simulink model "MultiUser_Model"  (R2016b)
settings: Solver=VariableStepAuto  StartTime=0.0  StopTime=inf  RelTol=1e-3
PreLoadFcn:
  | try, eval([bdroot '_setup']); catch, eval('MultiUser_setup', ''); end
libraries: MultiUser_Lib x3
settings Model: Creator=HP  LastModifiedBy=HP

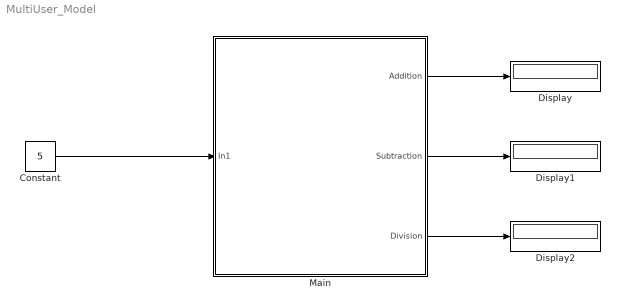
== system MultiUser_Model ==
  Constant : Constant  Value=5
  Display : Display
  Display1 : Display
  Display2 : Display
  Main : Subsystem
  wires:
  Constant/1 -> Main/1(In1)
  Main/1(Addition) -> Display/1
  Main/2(Subtraction) -> Display1/1
  Main/3(Division) -> Display2/1

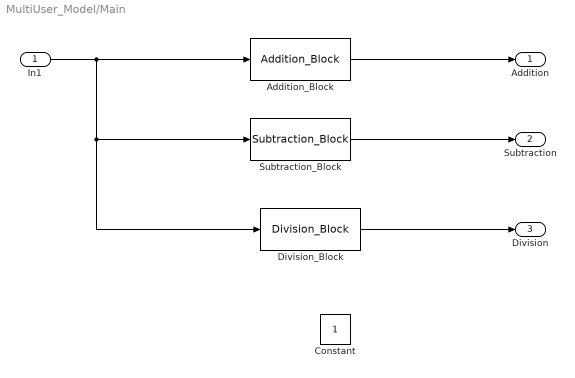
== system MultiUser_Model/Main ==
  In1 : Inport
  Addition_Block : MultiUser_Lib/Addition_Block
  Constant : Constant
  Division_Block : MultiUser_Lib/Division_Block
  Subtraction_Block : MultiUser_Lib/Subtraction_Block
  Addition : Outport
  Subtraction : Outport  Port=2
  Division : Outport  Port=3
  wires:
  In1/1 -> Addition_Block/1, Division_Block/1, Subtraction_Block/1
  Addition_Block/1 -> Addition/1
  Subtraction_Block/1 -> Subtraction/1
  Division_Block/1 -> Division/1
